simulink model "LKA_RL_training"  (R2022a)
settings: Solver=FixedStepAuto  StartTime=0.0  StopTime=T  FixedStep=Ts  RelTol=1e-3
undefined symbols (not defined in the file): Cf, Cr, DiscIntNeverNeededParam, e1_initial, e2_initial, isTerminate, Iz, lat_terminate_error, lf, lr, m, max_late_dev, max_rel_yaw_ang, md, rewardWeights, Ts, u_max, u_min, Vx
libraries: rllib x1, simulink x1
settings Model: Creator=The MathWorks, Inc.  LastModifiedBy=momentumlab
settings SolverCC: AlgebraicLoopSolver=TrustRegion
settings DataIOCC: ReturnWorkspaceOutputs=off
settings DebuggingCC: UnconnectedInputMsg=warning  UnconnectedOutputMsg=warning  UnconnectedLineMsg=warning  SFMachineParentedDataDiag=warning  ArithmeticOperatorsInVariantConditions=warning
settings SFSimCC: SimUseLocalCustomCode=off  CustomCodeUndefinedFunction=UseInterfaceOnly
settings RTWCC: RTWUseLocalCustomCode=off  DLArmComputeVersion=19.05
settings CodeAppCC: StateflowObjectComments=on
settings SimscapeCC: SimscapeNormalizeSystem=off

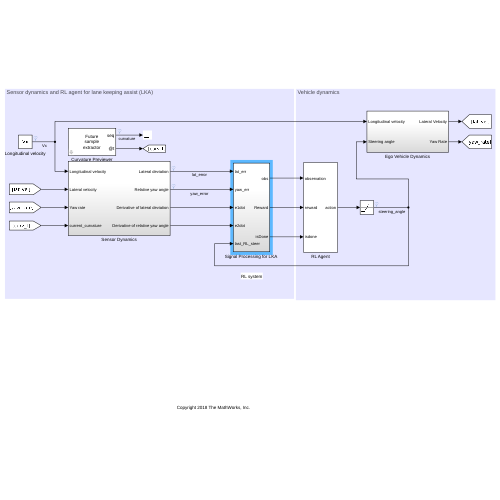
[thumbnail: Simulink's stored preview of the top-level diagram]
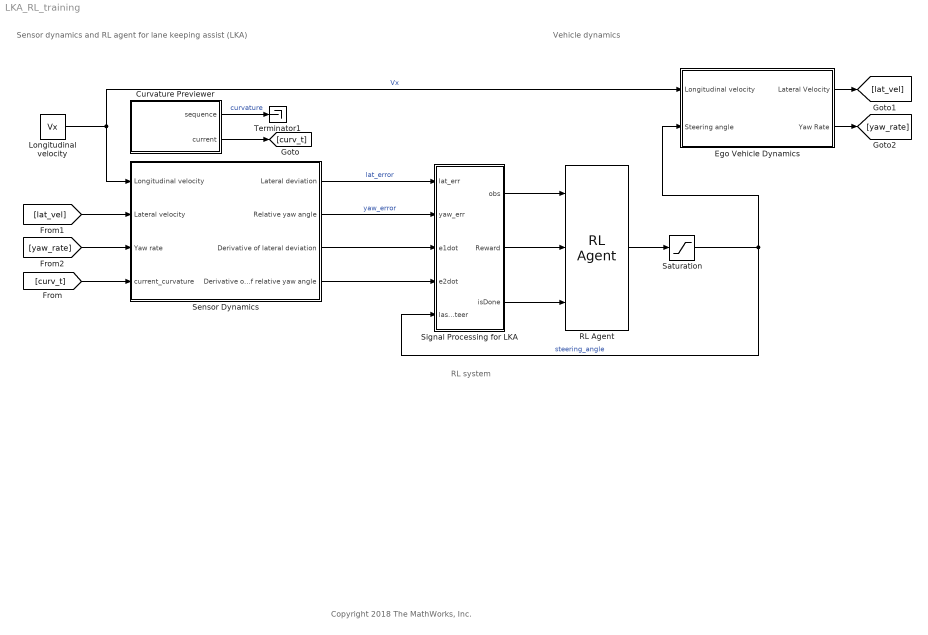
== system LKA_RL_training ==
  note: RL system
  note: Vehicle dynamics
  note: Sensor dynamics and RL agent for lane keeping assist (LKA)
  note: Copyright 2018 The MathWorks, Inc.
  Curvature Previewer : Subsystem  mask{signal=md, ts=Ts, steps=10}
      mask prompts: signal "Signal name"; ts "Sampling time"; steps "Number of previewing steps"
      mask init:
      | ts = evalin('base',get_param(gcbh,'ts'));
      | signal = evalin('base',get_param(gcbh,'signal'));
      | steps = evalin('base',get_param(gcbh,'steps'));
      | data = mpc_previewer_maskinit(signal,ts);
      mask Display:
      | fprintf('Future\nsample\nextractor');
      | port_label('output', 1, 'seq')
      | port_label('output', 2, '@t')
  Ego Vehicle Dynamics : Subsystem
  Longitudinal velocity : Constant  Value=Vx  SampleTime=Ts
  RL Agent : rllib/RL Agent  Agent=agent  ExternalActionAsInput=off  ProvideLastAction=off  ProvideCumRwd=off  TreatAsDirectFeedthrough=on  UseStrictObservationDataTypes=off
  Saturation : Saturate  UpperLimit=u_max  LowerLimit=u_min
  Sensor Dynamics : Subsystem
  "Signal Processing for LKA " : Subsystem
  Terminator1 : Terminator
  wires:
  Ego Vehicle Dynamics/1(Lateral Velocity) -> [lat_vel]
  Longitudinal velocity/1 -> Ego Vehicle Dynamics/1(Longitudinal velocity), Sensor Dynamics/1(Longitudinal velocity)  "Vx"
  Sensor Dynamics/1(Lateral deviation) -> "Signal Processing for LKA "/1(lat_err)  "lat_error"
  Sensor Dynamics/2(Relative yaw angle) -> "Signal Processing for LKA "/2(yaw_err)  "yaw_error"
  Sensor Dynamics/3(Derivative of lateral deviation) -> "Signal Processing for LKA "/3("e1dot ")
  Sensor Dynamics/4(Derivative of relative yaw angle) -> "Signal Processing for LKA "/4(e2dot)
  Curvature Previewer/2(current) -> [curv_t]
  [curv_t] -> Sensor Dynamics/4(current_curvature)
  Ego Vehicle Dynamics/2(Yaw Rate) -> [yaw_rate]
  [lat_vel] -> Sensor Dynamics/2(Lateral velocity)
  [yaw_rate] -> Sensor Dynamics/3(Yaw rate)
  "Signal Processing for LKA "/1(obs) -> RL Agent/1
  "Signal Processing for LKA "/2(Reward) -> RL Agent/2
  RL Agent/1 -> Saturation/1
  Saturation/1 -> "Signal Processing for LKA "/5(last_RL_steer), Ego Vehicle Dynamics/2(Steering angle)  "steering_angle"
  "Signal Processing for LKA "/3(isDone) -> RL Agent/3
  Curvature Previewer/1(sequence) -> Terminator1/1  "curvature"

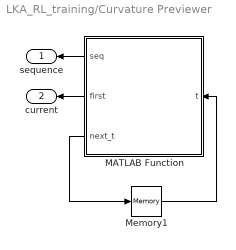
== system LKA_RL_training/Curvature Previewer ==
  MATLAB Function : MATLAB Function  TreatAsAtomicUnit=on
  Memory1 : Memory  InheritSampleTime=on  LinearizeAsDelay=on
  sequence : Outport  VectorParamsAs1DForOutWhenUnconnected=off
  current : Outport  Port=2  VectorParamsAs1DForOutWhenUnconnected=off
  wires:
  MATLAB Function/1(seq) -> sequence/1
  MATLAB Function/2(first) -> current/1
  Memory1/1 -> MATLAB Function/1(t)
  MATLAB Function/3(next_t) -> Memory1/1

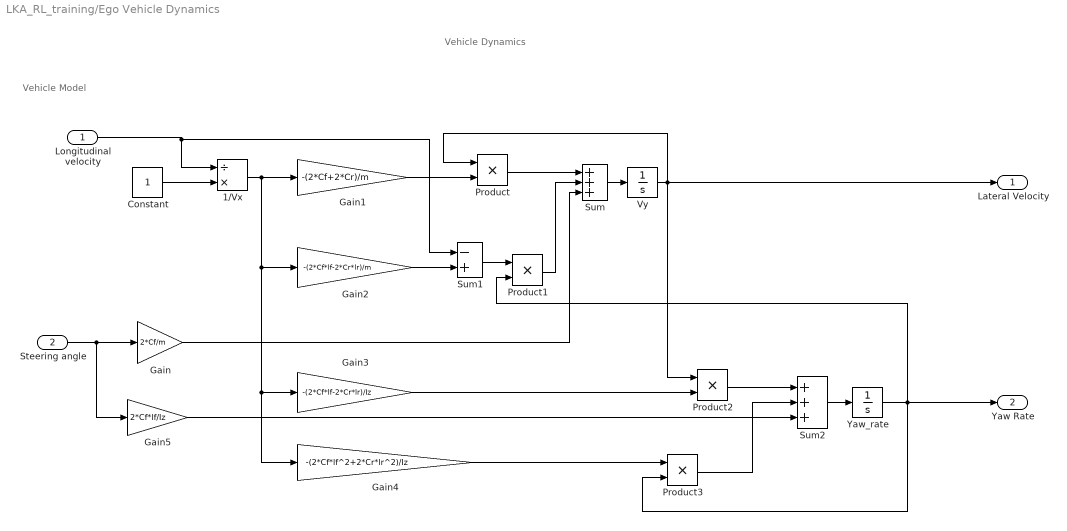
== system LKA_RL_training/Ego Vehicle Dynamics ==
  note: Vehicle Model
  note: Vehicle Dynamics
  Longitudinal velocity : Inport
  Steering angle : Inport  Port=2
  1/Vx : Product  Inputs=/*
  Constant : Constant
  Gain : Gain  Gain=2*Cf/m
  Gain1 : Gain  Gain=-(2*Cf+2*Cr)/m
  Gain2 : Gain  Gain=-(2*Cf*lf-2*Cr*lr)/m
  Gain3 : Gain  Gain=-(2*Cf*lf-2*Cr*lr)/Iz
  Gain4 : Gain  Gain=-(2*Cf*lf^2+2*Cr*lr^2)/Iz
  Gain5 : Gain  Gain=2*Cf*lf/Iz
  Product{,1..3} (4 alike) : Product
  Sum : Sum  Inputs=+++
  Sum1 : Sum  Inputs=-+
  Sum2 : Sum  Inputs=+++
  Vy : Integrator
  "Yaw_rate " : Integrator
  Lateral Velocity : Outport  VectorParamsAs1DForOutWhenUnconnected=off
  Yaw Rate : Outport  Port=2  VectorParamsAs1DForOutWhenUnconnected=off
  wires:
  Sum2/1 -> "Yaw_rate "/1
  Gain2/1 -> Sum1/2
  Gain4/1 -> Product3/1
  Constant/1 -> 1/Vx/2
  Gain3/1 -> Product2/2
  1/Vx/1 -> Gain4/1, Gain3/1, Gain2/1, Gain1/1
  Product2/1 -> Sum2/1
  Product3/1 -> Sum2/2
  Gain5/1 -> Sum2/3
  Sum1/1 -> Product1/1
  "Yaw_rate "/1 -> Product3/2, Yaw Rate/1, Product1/2
  Gain/1 -> Sum/3
  Steering angle/1 -> Gain/1, Gain5/1
  Gain1/1 -> Product/2
  Product/1 -> Sum/1
  Vy/1 -> Product/1, Lateral Velocity/1, Product2/1
  Sum/1 -> Vy/1
  Longitudinal velocity/1 -> Sum1/1, 1/Vx/1
  Product1/1 -> Sum/2

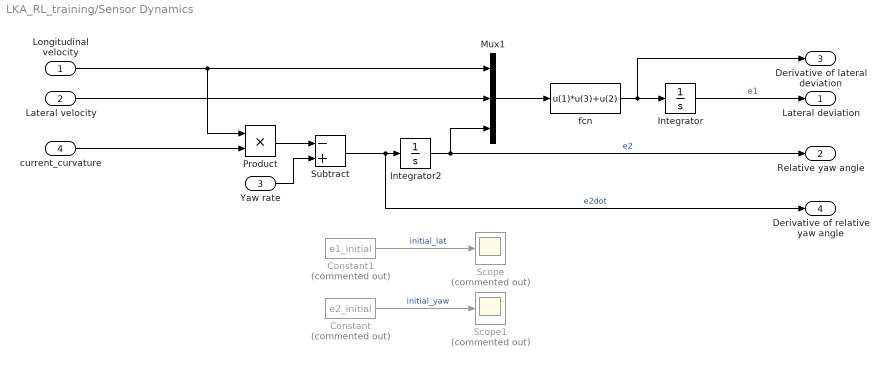
== system LKA_RL_training/Sensor Dynamics ==
  Longitudinal velocity : Inport
  Lateral velocity : Inport  Port=2
  Yaw rate : Inport  Port=3
  current_curvature : Inport  Port=4
  Constant : Constant  Commented=on  Value=e2_initial
  Constant1 : Constant  Commented=on  Value=e1_initial
  Integrator : Integrator  InitialCondition=e1_initial
  Integrator2 : Integrator  InitialCondition=e2_initial
  Mux1 : Mux  Inputs=[1 1 1]
  Product : Product
  Scope : Scope  Commented=on
  Scope1 : Scope  Commented=on
  Subtract : Sum  Inputs=-+
  fcn : Fcn  Expr=u(1)*u(3)+u(2)
  Lateral deviation : Outport  VectorParamsAs1DForOutWhenUnconnected=off
  Relative yaw angle : Outport  Port=2  VectorParamsAs1DForOutWhenUnconnected=off
  Derivative of lateral deviation : Outport  Port=3  VectorParamsAs1DForOutWhenUnconnected=off
  Derivative of relative yaw angle : Outport  Port=4  VectorParamsAs1DForOutWhenUnconnected=off
  wires:
  Integrator2/1 -> Relative yaw angle/1, Mux1/3  "e2"
  Mux1/1 -> fcn/1
  fcn/1 -> Derivative of lateral deviation/1, Integrator/1
  Lateral velocity/1 -> Mux1/2
  Integrator/1 -> Lateral deviation/1  "e1"
  Product/1 -> Subtract/1
  Yaw rate/1 -> Subtract/2
  Subtract/1 -> Derivative of relative yaw angle/1, Integrator2/1  "e2dot"
  Longitudinal velocity/1 -> Mux1/1, Product/1
  current_curvature/1 -> Product/2
  Constant1/1 -> Scope/1  "initial_lat"
  Constant/1 -> Scope1/1  "initial_yaw"

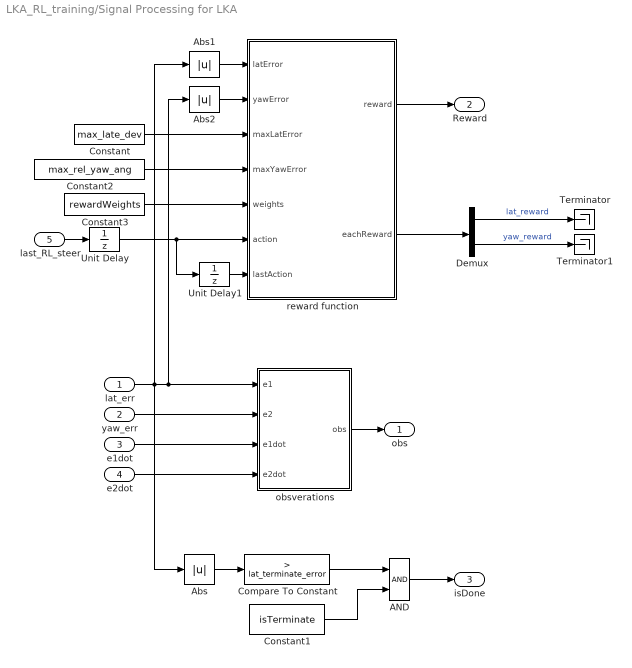
== system LKA_RL_training/Signal Processing for LKA  ==
  lat_err : Inport
  yaw_err : Inport  Port=2
  "e1dot " : Inport  Port=3
  e2dot : Inport  Port=4
  last_RL_steer : Inport  Port=5
  AND : Logic  IconShape=distinctive  AllPortsSameDT=off  OutDataTypeStr=boolean
  Abs : Abs  SaturateOnIntegerOverflow=off
  Abs1 : Abs  SaturateOnIntegerOverflow=off
  Abs2 : Abs  SaturateOnIntegerOverflow=off
  Compare To Constant : simulink/Logic and Bit Operations/Compare To Constant  relop=>  const=lat_terminate_error  OutDataTypeStr=boolean
  Constant : Constant  Value=max_late_dev
  Constant1 : Constant  Value=isTerminate
  Constant2 : Constant  Value=max_rel_yaw_ang
  Constant3 : Constant  Value=rewardWeights
  Demux : Demux  Outputs=2
  Terminator : Terminator
  Terminator1 : Terminator
  Unit Delay : UnitDelay  SampleTime=-1  HasFrameUpgradeWarning=on
  Unit Delay1 : UnitDelay  SampleTime=-1  HasFrameUpgradeWarning=on
  obsverations : Subsystem
  reward function : MATLAB Function  TreatAsAtomicUnit=on
  obs : Outport  VectorParamsAs1DForOutWhenUnconnected=off
  Reward : Outport  Port=2  VectorParamsAs1DForOutWhenUnconnected=off
  isDone : Outport  Port=3  VectorParamsAs1DForOutWhenUnconnected=off
  wires:
  obsverations/1(obs) -> obs/1
  "e1dot "/1 -> obsverations/3(e1dot)
  e2dot/1 -> obsverations/4(e2dot)
  yaw_err/1 -> obsverations/2(e2)
  lat_err/1 -> obsverations/1(e1), Abs2/1, Abs1/1, Abs/1
  reward function/1(reward) -> Reward/1
  Constant/1 -> reward function/3(maxLatError)
  Abs1/1 -> reward function/1(latError)
  Abs2/1 -> reward function/2(yawError)
  last_RL_steer/1 -> Unit Delay/1
  Abs/1 -> Compare To Constant/1
  Compare To Constant/1 -> AND/1
  Constant1/1 -> AND/2
  AND/1 -> isDone/1
  Constant3/1 -> reward function/5(weights)
  Unit Delay1/1 -> reward function/7(lastAction)
  Constant2/1 -> reward function/4(maxYawError)
  Unit Delay/1 -> Unit Delay1/1, reward function/6(action)
  reward function/2(eachReward) -> Demux/1
  Demux/1 -> Terminator/1  "lat_reward"
  Demux/2 -> Terminator1/1  "yaw_reward"

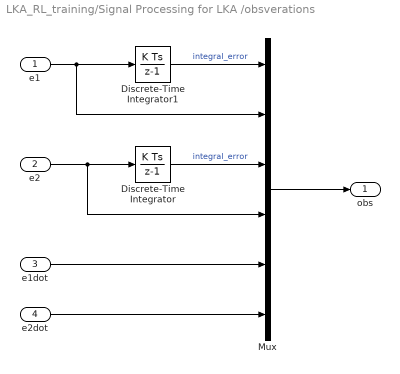
== system LKA_RL_training/Signal Processing for LKA /obsverations ==
  e1 : Inport
  e2 : Inport  Port=2
  e1dot : Inport  Port=3
  e2dot : Inport  Port=4
  Discrete-Time Integrator : DiscreteIntegrator  SampleTime=-1  ICPrevOutput=DiscIntNeverNeededParam  ICPrevScaledInput=DiscIntNeverNeededParam
  Discrete-Time Integrator1 : DiscreteIntegrator  SampleTime=-1  ICPrevOutput=DiscIntNeverNeededParam  ICPrevScaledInput=DiscIntNeverNeededParam
  Mux : Mux  Inputs=6
  obs : Outport  VectorParamsAs1DForOutWhenUnconnected=off
  wires:
  e1/1 -> Mux/2, Discrete-Time Integrator1/1
  Mux/1 -> obs/1
  Discrete-Time Integrator1/1 -> Mux/1  "integral_error"
  e2/1 -> Mux/4, Discrete-Time Integrator/1
  Discrete-Time Integrator/1 -> Mux/3  "integral_error"
  e1dot/1 -> Mux/5
  e2dot/1 -> Mux/6

== matlab function LKA_RL_training/Signal Processing for LKA /reward function ==
  data: latError input; reward output; yawError input; maxLatError input; maxYawError input; weights input; action input; lastAction input; eachReward output
function [reward,eachReward] = fcn(latError, yawError, maxLatError, maxYawError, weights, action, lastAction)


if latError <= maxLatError
    latReward = tanh(3*abs(maxLatError-latError));
else
    latReward = -tanh(3*abs(maxLatError-latError));
end


if yawError <= maxYawError
    yawReward = tanh(8*abs(maxYawError-yawError));
else
    yawReward = -tanh(9*abs(maxYawError-yawError));
end

stepReward = 0.05;
stableReward = -(action-lastAction)^2;

reward = weights(1)*latReward + weights(2)*yawReward + weights(3)*stableReward + stepReward;
eachReward = [latReward,yawReward];

== matlab function LKA_RL_training/Curvature Previewer/MATLAB Function ==
  settings: updateMethod=DISCRETE  sampleTime=ts
  data: data parameter; seq output; steps parameter; t input; first output; next_t output
function [seq,first,next_t] = fcn(data,steps,t)
%#codegen
[seq,first,next_t] = mpcblock_preview('md',data,steps,t);
